simulink model "PlantIdentification"  (R2025b)
settings: Solver=ode14x  StartTime=0.0  StopTime=2 * (seqLen * Ts_ctrl)  FixedStep=Ts_local  RelTol=1e-3
model workspace (MAT data in the model file):
  GateChoice = "linear"
  seqLen = 511
  seqW = 1
undefined symbols (not defined in the file or in its folder): Ts_ctrl, u_b
libraries: simulink x1
settings Model: DataDictionary=ctrlSys.sldd  SimulationMode=accelerator  Creator=LYG  LastModifiedBy=A

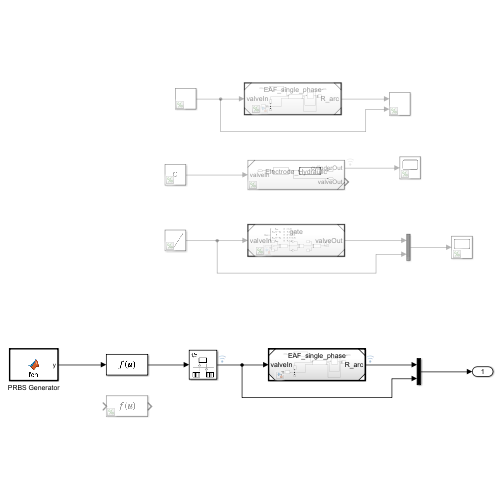
[thumbnail: Simulink's stored preview of the top-level diagram]
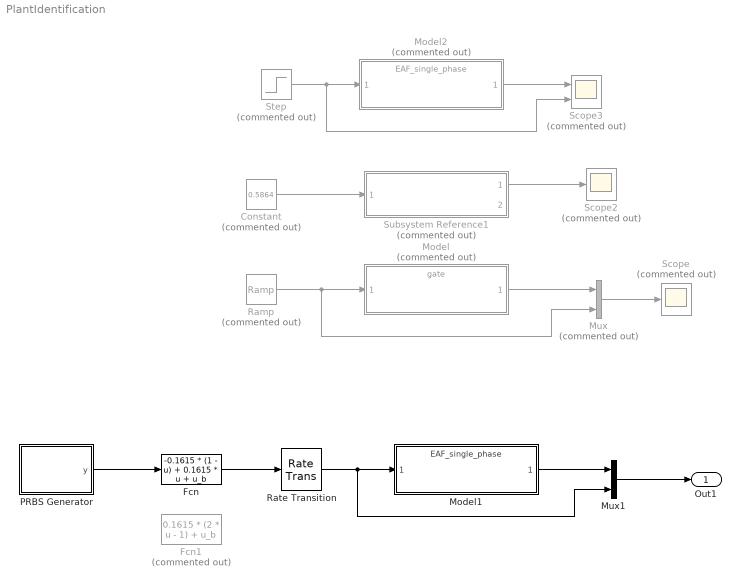
== system PlantIdentification ==
  Constant : Constant  Commented=on  Value=0.5864
  Fcn : Fcn  Expr=-0.1615 * (1 - u) + 0.1615 * u + u_b
  Fcn1 : Fcn  Commented=on  Expr=0.1615 * (2 * u - 1) + u_b
  Model : ModelReference  Commented=on  ModelNameDialog=gate.slx  SimulationMode=Normal  ModelReferenceVersion=3.11
  Model1 : ModelReference  ModelNameDialog=EAF_single_phase.slx  SimulationMode=Normal  ModelReferenceVersion=1.21
  Model2 : ModelReference  Commented=on  ModelNameDialog=EAF_single_phase.slx  SimulationMode=Normal  ModelReferenceVersion=1.20
  Mux : Mux  Commented=on  Inputs=2
  Mux1 : Mux  Inputs=2
  PRBS Generator : MATLAB Function  TreatAsAtomicUnit=on  SystemSampleTime=Ts_ctrl
  Ramp : simulink/Sources/Ramp  Commented=on  slope=0.4  start=0  InitialOutput=-2
  Rate Transition : RateTransition  InitialCondition=u_b  OutPortSampleTime=Ts_local
  Scope : Scope  Commented=on
      settings: ActiveDisplayYMinimum=-0.00525  ActiveDisplayYMaximum=0.0072499999999999995
  Scope2 : Scope  Commented=on
      settings: ActiveDisplayYMinimum=-0.00525  ActiveDisplayYMaximum=0.0072499999999999995  DataLoggingVariableName=ScopeData2
  Scope3 : Scope  Commented=on  NumInputPorts=2
      settings: ActiveDisplayYMinimum=-0.003033654025755771  ActiveDisplayYMaximum=0.027302886231801948  DataLoggingVariableName=ScopeData3
  Step : Step  Commented=on  Before=u_b  After=u_b + 0.168  SampleTime=0
  Subsystem Reference1 : Subsystem  Commented=on  ReferencedSubsystem=Electrode_Hydraulic
  Out1 : Outport
  wires:
  Ramp/1 -> Mux/2, Model/1
  Model/1 -> Mux/1
  Mux/1 -> Scope/1
  PRBS Generator/1(y) -> Fcn/1
  Model1/1 -> Mux1/1
  Mux1/1 -> Out1/1
  Fcn/1 -> Rate Transition/1
  Rate Transition/1 -> Mux1/2, Model1/1
  Constant/1 -> Subsystem Reference1/1
  Subsystem Reference1/1 -> Scope2/1
  Model2/1 -> Scope3/1
  Step/1 -> Scope3/2, Model2/1

== matlab function PlantIdentification/PRBS Generator ==
  data: y output; seqLen parameter size=[1 1]; seqW parameter size=[1 1]
function y = fcn(seqLen, seqW)
% Codegen-friendly PRBS using an LFSR (max-length).
% Output levels: {0,1}. Each bit is held for seqW samples.

persistent lfsr m hold

if isempty(lfsr)
    % Choose LFSR order so period >= seqLen
    m = max(2, ceil(log2(double(seqLen) + 1)));
    if m > 16
        m = 16; % limit to supported taps below
    end
    lfsr = uint32(1); % non-zero seed
    hold = uint32(0);
end

% Advance LFSR only when hold counter expires
if hold == 0
    fb = lfsr_feedback(lfsr, m);
    lfsr = bitshift(lfsr, 1);
    lfsr = bitset(lfsr, 1, fb);
    lfsr = bitand(lfsr, bitshift(uint32(1), m) - 1);
    hold = uint32(max(1, seqW)); % hold each bit for seqW samples
end

y = double(bitget(lfsr, 1));
hold = hold - 1;

end

function fb = lfsr_feedback(s, m)
% Max-length taps for m = 2..16 (Fibonacci form)
switch m
    case 2
        fb = bitxor(bitget(s,2), bitget(s,1));
    case 3
        fb = bitxor(bitget(s,3), bitget(s,2));
    case 4
        fb = bitxor(bitget(s,4), bitget(s,3));
    case 5
        fb = bitxor(bitget(s,5), bitget(s,3));
    case 6
        fb = bitxor(bitget(s,6), bitget(s,5));
    case 7
        fb = bitxor(bitget(s,7), bitget(s,6));
    case 8
        fb = bitxor(bitxor(bitget(s,8), bitget(s,6)), bitxor(bitget(s,5), bitget(s,4)));
    case 9
        fb = bitxor(bitget(s,9), bitget(s,5));
    case 10
        fb = bitxor(bitget(s,10), bitget(s,7));
    case 11
        fb = bitxor(bitget(s,11), bitget(s,9));
    case 12
        fb = bitxor(bitxor(bitget(s,12), bitget(s,6)), bitxor(bitget(s,4), bitget(s,1)));
    case 13
        fb = bitxor(bitxor(bitget(s,13), bitget(s,4)), bitxor(bitget(s,3), bitget(s,1)));
    case 14
        fb = bitxor(bitxor(bitget(s,14), bitget(s,5)), bitxor(bitget(s,3), bitget(s,1)));
    case 15
        fb = bitxor(bitget(s,15), bitget(s,14));
    otherwise % 16
        fb = bitxor(bitxor(bitget(s,16), bitget(s,15)), bitxor(bitget(s,13), bitget(s,4)));
end
end
